simulink model "cursorTask"  (R2012b)
settings: Solver=FixedStepDiscrete  StartTime=0.0  StopTime=10.0  FixedStep=0.001  RelTol=1e-3
undefined symbols (not defined in the file): acquireMethods, autoplayMovementDuration, autoplayReactionTime, autoplayRotationDuration, autoplayRotationStart, centerOffset, clickPercentage, clickRefractoryPeriod, clickTargetColor, clickTargetHoverColor, clickTargs, coherences, contextIDs, contextTime, contextTimeVec, crossSize, cuedText, cuedTextLength, cumulativeDwell, cursorColorClick, cursorColorClosed, cursorColorOpen, cursorColors, cursorDiameter, cursorNeuralColor, cursorNonneuralColor, delayOrder, delayPeriodGainScale, delayTime, discreteOLMode, displayObject, doHeadSpeedFail, drawNumbersOnTargets, dwellRefractoryPeriod, errorAssistAxis, errorAssistR, errorAssistTheta, expRandBinSize, expRandMax, expRandMin, expRandMu, eyeMode, failOnLiftoff, failurePenalty, falseClickFails, fingerPositionTolerance, fixedSeqMode, freePlayMode, gain, gloveBias, gloveLPDenominator, gloveLPNumerator, gloveNonlinearCorrection, gloveXCorrection, gloveYCorrection, gracePeriod, gridEdges, gridSize, gridTilesEachDim, headSpeedCap ... (+134)
(part 2 of 2)

== matlab function cursorTask/cursorTaskSplit ==
  data: xkRaw input double size=[double(xkConstants.NUM_STATE_DIMENSIONS) 1]; xkMod input; behaviorPacket input Bus: behaviorPacketBus size=1; vizData input Bus: peripheralData; clickState input; clickParameters input; taskOutput output Bus: taskOutput; stateParameters input Bus: stateParams size=1; cursorParameters input Bus: taskParamsBus; clock input; xpcTET input; xkModBiasEst input; taskAgnosticXk input; xkAux input
function taskOutput  = cursorTaskCerebus(xkRaw, xkMod, behaviorPacket, vizData, clickState, clickParameters, ...
    stateParameters, cursorParameters, clock, xpcTET, xkModBiasEst, taskAgnosticXk, xkAux)
%#codegen
% This is the state-machine-like implementation of the cursor task. 
% This, depending on paraemters, can do center-out-and-back
%
% October 31 2016: now has two state inputs, xkRaw (which gets fed back to
% the decoder), and xkMod. Generally should look at xkMod for task logic,
% but if the game needs to change a state element which ought to propogate
% into the decoder (for example re-seed the cursor), it should do this to
% both xkRaw and xkMod.

% cursorParameters is actually taskParamsBus, which is set by
% cursotTask_buildWorkspace.m

mouse = behaviorPacket.mouse(1:6);
glove = behaviorPacket.glove(1:5);
robotPosition = behaviorPacket.robotPosition; % 1x3 of x y z % SDS I *think* but need to check that this is the returned position of robot
behaviorRequestClock = behaviorPacket.xpcRequestClock;
peripheralTimestamp = behaviorPacket.peripheralTimestamp(1:16);
%% CONSTANTS
TASK_NAME = 'cursor';
VERSION_ID = single(3.13); % updated to 3.13 with MULTICLICK task -SF
% looking at TASK_DIMS instead of NUM_DIMS to 5D % DIMENSION-DEPENDENT
% NUM_DIMS is dimensionality as the task code was compiled. August 2016 raised this from 2 to 3. Feb 2017 took this to 4
% Actual task can use fewer dimensions, e.g. running 4D with a 5D
% compilation. Look to TASK_DIMS for that. It is defined from locked
% parameters down below
NUM_DIMS = uint8(cursorConstants.NUM_DIMENSIONS); % 
INIT_LENGTH = uint16(100); %ms
% PRE_TRIAL_LENGTH = uint16(20); %ms
SCORE_LENGTH = uint16(4000); %ms
INIT_TIME = uint32(2000);

cursorPosition2 = single( nan(1,NUM_DIMS) ); % Aux cursor and used for RAYS. Can send a second cursor position.
cursorAlpha2 = uint8(100); % used for RAYS, otherwise 100. This is in %.
%% INITIALIZE FILELOGGER DATA
fileLoggerData.data = uint8(zeros(1,1400));
fileLoggerData.dataLen = uint16(0);
fileLoggerData.fileName = uint8(zeros(1,20));
fileLoggerData.send = false;

fileLoggerFormat.format = uint8(zeros(1,1400));
fileLoggerFormat.formatLen = uint16(0);
fileLoggerFormat.fileName = uint8(zeros(1,20));

fileLoggerFormatAndData.format = fileLoggerFormat;
fileLoggerFormatAndData.data = fileLoggerData;
%% INITIALIZE CURSOR TASK OUTPUT - DO NOT REMOVE ANY ASSIGNMENTS, ORDER MATTERS
allowStop = true;
resetHMM = false;

taskOutput.flushFiles = false;
taskOutput.sendFormat = false;
taskOutput.taskDetails = fileLoggerFormat;
taskOutput.discrete = fileLoggerFormatAndData;
taskOutput.continuous = fileLoggerFormatAndData;
taskOutput.screen = fileLoggerFormatAndData;
taskOutput.sound = fileLoggerFormatAndData;
taskOutput.asynch = fileLoggerFormatAndData;
taskOutput.ttl = double(0);
taskOutput.xk = xkRaw;
taskOutput.inputType = cursorParameters.initialInput;
taskOutput.currentTarget = single(zeros([double(xkConstants.NUM_TARGET_DIMENSIONS) 1]));
taskOutput.state = uint16(CursorStates.STATE_INIT);
taskOutput.paused = false;
taskOutput.allowStop = allowStop;
taskOutput.resetHMM = resetHMM;
taskOutput.wiaCode = uint16(1); %garbage
taskOutput.speedCode = uint16(1); %garbage
taskOutput.clickTarget = uint16(DiscreteStates.CLICK_IDLE); 
taskOutput.taskType = uint16(cursorConstants.TASK_CENTER_OUT); %default value -SNF
%% TASK DETAILS PACKET
taskOutput.taskDetails = packFileLoggerTaskDetails(TASK_NAME, VERSION_ID, ...
    'STATE_INIT', uint8(CursorStates.STATE_INIT), ...
    'STATE_PRE_TRIAL', uint8(CursorStates.STATE_PRE_TRIAL),...
    'STATE_NEW_TARGET', uint8(CursorStates.STATE_NEW_TARGET),...
    'STATE_MOVE', uint8(CursorStates.STATE_MOVE),...
    'STATE_ACQUIRE', uint8(CursorStates.STATE_ACQUIRE),...
    'STATE_SUCCESS', uint8(CursorStates.STATE_SUCCESS),...
    'STATE_FAIL', uint8(CursorStates.STATE_FAIL),...
    'STATE_CENTER_TARGET', uint8(CursorStates.STATE_CENTER_TARGET),...
    'STATE_END', uint8(CursorStates.STATE_END),...
    'STATE_RECENTER_DELAY', uint8(CursorStates.STATE_RECENTER_DELAY),...
    'STATE_MOVE_CLICK', uint8(CursorStates.STATE_MOVE_CLICK),...
    'STATE_MOVE_HOVER', uint8(CursorStates.STATE_HOVER),... %SNF: Why in the actual f is this named move_hover and then mapped to just hover??? 
    'STATE_FINGER_MOVED', uint8(CursorStates.STATE_FINGER_MOVED),...
    'CLICK_IDLE', uint8(DiscreteStates.CLICK_IDLE),...
    'CLICK_MAIN', uint8(DiscreteStates.CLICK_MAIN),...
    'TARGET_TYPE_DWELL', uint8(cursorConstants.TARGET_TYPE_DWELL), ...
    'TARGET_TYPE_CLICK', uint8(cursorConstants.TARGET_TYPE_CLICK), ...
    'INPUT_TYPE_MOUSE_ABSOLUTE', uint8(cursorConstants.INPUT_TYPE_MOUSE_ABSOLUTE),...
    'INPUT_TYPE_DECODE_V', uint8(cursorConstants.INPUT_TYPE_DECODE_V),...
    'INPUT_TYPE_AUTO_PLAY', uint8(cursorConstants.INPUT_TYPE_AUTO_PLAY),...
    'CLICK_TYPE_NONE', uint8(clickConstants.CLICK_TYPE_NONE),...
    'CLICK_TYPE_GLOVE', uint8(clickConstants.CLICK_TYPE_GLOVE),...
    'CLICK_TYPE_NEURAL', uint8(clickConstants.CLICK_TYPE_NEURAL),...
    'OUTPUT_TYPE_CURSOR', uint8(cursorConstants.OUTPUT_TYPE_CURSOR),...
    'OUTPUT_TYPE_ROBOT', uint8(cursorConstants.OUTPUT_TYPE_ROBOT)...
);
%% DEFINE PERSISTENTS
persistent state vizPacket;
persistent pauseTriggered;
persistent stateTimer;
persistent holdTimer;
persistent clickTimer; %added SDS Jan 2017, so both click and hold can be used to do this task
persistent cursorColors;
persistent targetRadiusTrans % added SDS Feb 2017, this is the target radius in XYZ
persistent targetRadiusRot % added SDS Feb 2017, this is the target radius in rotation
persistent currentTarget;
persistent nextTarget;
persistent nextClickTarg currentClickTarg; %SNF multiclick
persistent speedCode;
persistent wiaCode;
% below are used for gridlike task, which divides workspace into tiles and
% fails if dwell or click over wrong tile (which makes it a lot like grid
% task. SDS Dec 2016
% D refers to xkConstants.NUM_TARGET_DIMENSIONS, but really not all might
% be used; lockedParams.gridTilesEachDim specifies which dimensions are
% active and how many tiles each dimension is divided into
persistent currentTargetTile; % D x 1 vector of indices into lockedParams.gridEdges. Current active tile I want to go to
persistent nextTargetTile; % D x 1 vector of indices into lockedParams.gridEdges. What the next active target tile will be
persistent currentOccupiedTile; % D x 1 vector of indices specying which tile is currently being occupied.
persistent previousOccupiedTile; % D x 1 vector of indicies specifying which tile was occupied in the previous time step.

persistent currentTargetType nextTargetType;  % dwell or click
persistent trialNum targetOrder cycleNum cycleIndex;
persistent trialDelayLength;

persistent localAcquired localTotal localTotalTime localAcqTime;
persistent localScore totalScore;
persistent acquireTime lastState;

persistent lockedParameters inputType outputType;
persistent stateBeforePreTrial;

persistent lastSoundTime;
persistent lastSoundState;

persistent initialFingerPosition initialCursorPosition previousInput;

persistent totalTaskTime;
persistent lastAcquireSuccess previousTarget;

persistent filteredHeadSpeed;
persistent prevHeadPos;
persistent lastHeadSpeedFail;
%SNF mulitclick: 
persistent prevClickState; 
persistent multiClickColors; 
%% INITIALIZE PERSISTENTS
if(isempty(state))
    state = uint16(CursorStates.STATE_INIT);
    lastState = state;
    currentTarget = single(zeros([double(xkConstants.NUM_TARGET_DIMENSIONS) 1]));
    nextTarget = single(zeros([double(xkConstants.NUM_TARGET_DIMENSIONS) 1]));
    currentTargetTile = uint16(zeros([double(xkConstants.NUM_TARGET_DIMENSIONS) 1])); % SDS Dec 2016
    nextTargetTile = uint16(zeros([double(xkConstants.NUM_TARGET_DIMENSIONS) 1])); % SDS Dec 2016
    currentOccupiedTile = uint16(zeros([double(xkConstants.NUM_TARGET_DIMENSIONS) 1])); % SDS Dec 2016
    previousOccupiedTile = uint16(zeros([double(xkConstants.NUM_TARGET_DIMENSIONS) 1])); % SDS Dec 2016
   
    speedCode = uint16(0); %FRW hacky instructed speed experiment
    wiaCode = uint16(0); %FRW hacky wia experiment
    nextClickTarg = uint16(0);  %SNF for identifying which click target to use
    currentClickTarg = uint16(0);
    
    vizPacket = initVizPacket;
    stateTimer = uint16(0);
    holdTimer = int16(0);
    clickTimer = int16(0); % initialize
    pauseTriggered = true;
    
    cursorColors = double(zeros([3 3])); % there's a second cursor (column 2) allowed; now a third for eye cursor 
    filteredHeadSpeed = single(0);
    prevHeadPos = single(zeros(2,1));

    targetOrder = uint16(ones([1 double(cursorConstants.MAX_TARGETS)]));
    trialNum = uint16(0);
    cycleNum = uint16(0);
    cycleIndex = uint16(1); % 1 so it's a valid idnex even when first used
    trialDelayLength = uint16(0);
    
    localTotal = uint16(0);
    localTotalTime = uint16(0);
    localAcquired = uint16(0);
    localAcqTime = uint16(0);
    localScore = uint16(0);
    totalScore = uint16(0);
    acquireTime = stateTimer;
    currentTargetType = uint16(cursorConstants.TARGET_TYPE_DWELL);
    nextTargetType = uint16(cursorConstants.TARGET_TYPE_DWELL);
	stateBeforePreTrial = uint16(0);
    lastSoundTime = clock;
    lastSoundState = uint8(CursorStates.SOUND_STATE_IDLE);
    
    initialFingerPosition = mouse(1:2);
    initialCursorPosition = single( zeros(NUM_DIMS,1) );
    
    totalTaskTime = uint32(0);
    lastHeadSpeedFail = uint32(0);
    
    lastAcquireSuccess = false;
    previousTarget = currentTarget;
    prevClickState =  uint16(DiscreteStates.CLICK_IDLE); %upon starting, intiialize to not clicking 
        %% buffer all the parameters off the bus
    lockedParameters = cursorParameters;
    targetRadiusTrans = double(lockedParameters.targetDiameter) / 2;
    targetRadiusRot = double(lockedParameters.targetRotDiameter) / 2;
    inputType = lockedParameters.initialInput;
    multiClickColors =  single(lockedParameters.multiclickColors); % single([[255 24 29];[255 0 255]; [140 150 198]; [0 102 255]]); %SNF multiclick- hard coding for now, make this a matrix in task doc
%%
    previousInput = inputType;
end
%% some initialization
if(clock < INIT_TIME)
    pauseTriggered = true;
end
outputType = cursorParameters.outputType; % determines what graphics engine will render this task.
% We usually shouldn't write discrete data
writeDiscreteData = false;
writeContinuousData = true;

if(vizData.receive && (vizData.dataLen > 0 ))
    vizPacket = parseVizPacket(vizData.data);
end

isNeural = (uint16(inputType) == uint16(cursorConstants.INPUT_TYPE_DECODE_V));
%isClicked = (uint16(clickState) == uint16(DiscreteStates.CLICK_MAIN)); %SF: this needs to be more flexible
isClicked = (uint16(clickState) >= uint16(DiscreteStates.CLICK_MAIN)); %SF: this includes multiclick options
isNone = (uint16(inputType) == uint16(cursorConstants.INPUT_TYPE_NONE));
if clickTimer < 0
    clickTimer = clickTimer + 1; %always counts up while negative, thus using up refractory period
end
% clickTimer counts up only in certain states (i.e. only certain states
% allow click accumulation).
if ~isClicked && clickTimer > 0 % doesn't reset to zero when in refractory period.
    clickTimer = int16(0); % resets to be not-clicked
end
%% set the cursor color 
% SNF: add different colors for different clicks in multiclick 
if isClicked
    if uint16(lockedParameters.taskType) == uint16(cursorConstants.TASK_MULTICLICK)
        cursorColors(1:end, 1) = multiClickColors(uint16(clickState-1), 1:end); 
    else
        cursorColors(1:end,1) = lockedParameters.cursorColorClick; %[255; 0; 0;];
    end
elseif isNeural
    cursorColors(1:end,1) = [255; 255; 255;];
elseif isNone
    cursorColors(1:end,1) = [0; 204; 102;];
elseif uint16(inputType) == uint16(cursorConstants.INPUT_TYPE_HEAD_MOUSE)
    cursorColors(1:end,1) = [0; 204; 102;]; %head position is always green
elseif uint16(inputType) == uint16(cursorConstants.INPUT_TYPE_HEAD_CURSORSTILL)
    cursorColors(1:end,1) = [0; 204; 102;]; %primary color represents head position so color it green
else % This is used for autoplay.
    cursorColors(1:end,1) = [255; 255; 255]; % 
%     cursorColors(1:end,1) = [200; 255; 200]; % slightly minty % SDS April 2017: T5 hates minty color, just making it white
end
% these are default colors, individual states can overwrite if they want.
switch lockedParameters.taskType
    case  uint32(cursorConstants.TASK_GRIDLIKE)
        targetColor = 'a'; % in gridlike, target is aqua
    otherwise
        targetColor = 'a'; % in other tasks, target still aqua
end
%% %WIA stuff
if (uint16(lockedParameters.wiaMode) == uint16(cursorConstants.WIA_IMAGINE_ONLY)) || ...
        (uint16(lockedParameters.wiaMode) == uint16(cursorConstants.WIA_IMAGINE_ONLY_NO_HC))
    wiaCode = uint16(2);
elseif uint16(lockedParameters.wiaMode) == uint16(cursorConstants.WIA_WATCH_ONLY)
    wiaCode = uint16(1);
elseif uint16(lockedParameters.wiaMode) == uint16(cursorConstants.WIA_DO_ONLY)
    wiaCode = uint16(3);
end
%% which state elements do I look to for the cursor's position? SDS July 2016
xk2HorizontalPos = uint8( lockedParameters.xk2HorizontalPos );
xk2VerticalPos = uint8( lockedParameters.xk2VerticalPos );
xk2HorizontalVel = uint8( lockedParameters.xk2HorizontalVel );
xk2VerticalVel = uint8( lockedParameters.xk2VerticalVel );
xk2DepthPos = uint8( lockedParameters.xk2DepthPos );
xk2DepthVel = uint8( lockedParameters.xk2DepthVel );
xk2RotatePos = uint8( lockedParameters.xk2RotatePos );
xk2RotateVel = uint8( lockedParameters.xk2RotateVel );
xk2Rotate2Pos = uint8( lockedParameters.xk2Rotate2Pos );
xk2Rotate2Vel = uint8( lockedParameters.xk2Rotate2Vel );
% DIMENSION-DEPENDENT
TASK_DIMS = lockedParameters.numDisplayDims; % only used for determining what kind of
% checking to use. We still need to have everything be NUM_DIMS long or
% things won't compile.
canBePosInds = [xk2HorizontalPos,xk2VerticalPos,xk2DepthPos,xk2RotatePos,xk2Rotate2Pos];
canBeVelInds = [xk2HorizontalVel,xk2VerticalVel,xk2DepthVel,xk2RotateVel,xk2Rotate2Vel];
effectorPosInds = canBePosInds(1:NUM_DIMS);
effectorVelInds = canBeVelInds(1:NUM_DIMS);

if uint16(inputType) == uint16(cursorConstants.INPUT_TYPE_HEAD_CURSORSTILL)
    effectorPos = xkAux(effectorPosInds);
    effectorVel = xkAux(effectorVelInds);
    auxEffectorPos = xkMod(effectorPosInds);
    displayAuxCursor = true;
    cursorColors(1:end,2) = [255; 255; 255];
elseif uint16(inputType) == uint16(cursorConstants.INPUT_TYPE_CURSOR_HEADSTILL) || ...
        uint16(inputType) == uint16(cursorConstants.INPUT_TYPE_AUTO_ACQUIRE_HS)
    effectorPos = xkMod(effectorPosInds);
    effectorVel = xkMod(effectorVelInds);
    auxEffectorPos = xkAux(effectorPosInds);
    displayAuxCursor = true;
    cursorColors(1:end,2) = [0; 204; 102;];
elseif uint16(inputType) == uint16(cursorConstants.INPUT_TYPE_CURSOR_AND_HEAD)
    effectorPos = xkMod(effectorPosInds);
    effectorVel = xkMod(effectorVelInds);
    %for target acquisiotn logic, the 3rd and 4th dimensions of the cursor
    %will be equal to auxiliary cursor X and Y and the task will be 4-dimensional
    effectorPos(3:4) = xkAux(effectorPosInds(1:2));
    effectorVel(3:4) = xkAux(effectorVelInds(1:2));
    auxEffectorPos = xkAux(effectorPosInds);
    displayAuxCursor = true;
    cursorColors(1:end,2) = [0; 204; 102;];
elseif uint16(inputType) == uint16(cursorConstants.INPUT_TYPE_WIA_HEAD)
    if wiaCode==uint16(1) || wiaCode==uint16(2) %watch, imagine
        effectorPos = xkMod(effectorPosInds);
        effectorVel = xkMod(effectorVelInds);
        auxEffectorPos = xkAux(effectorPosInds);
        if (uint16(lockedParameters.wiaMode) == uint16(cursorConstants.WIA_IMAGINE_ONLY_NO_HC))
            displayAuxCursor = false;
        else
            displayAuxCursor = true;
        end
        cursorColors(1:end,2) = [0; 204; 102;];
    else %attempt
        effectorPos = xkAux(effectorPosInds);
        effectorVel = xkAux(effectorVelInds);
        auxEffectorPos = xkMod(effectorPosInds);
        displayAuxCursor = false;
        cursorColors(1:end,1) = [0; 204; 102;];
    end
else
    effectorPos = xkMod(effectorPosInds);
    effectorVel = xkMod(effectorVelInds);
    auxEffectorPos = zeros(NUM_DIMS,1);
    displayAuxCursor = false;
end
%% %head speed check; we low pass filter the 1ms head speed and can fail the trial if it is too high
headSpeedAlpha = single(0.96);
headSpeed = 1000*sqrt(sum((behaviorPacket.windowsMousePosition - prevHeadPos).^2));
filteredHeadSpeed = headSpeedAlpha*filteredHeadSpeed + (1-headSpeedAlpha)*headSpeed;
prevHeadPos = behaviorPacket.windowsMousePosition;
%fail if moving the head when he shouldn't be
if (lockedParameters.doHeadSpeedFail || wiaCode==uint16(1) || wiaCode==uint16(2)) && (filteredHeadSpeed > lockedParameters.headSpeedCap) ...
    &&((clock - lastHeadSpeedFail)>2000)
    %stateTimer = uint16(0);
    %state = uint16(CursorStates.STATE_FAIL);
    lastHeadSpeedFail = clock;
    lastSoundTime = clock;
    lastSoundState = uint8(CursorStates.SOUND_STATE_FAIL);
end
%% %really hacky eye mode
eyePos = behaviorPacket.windowsPC1GazePoint;
eyePos(1) = (eyePos(1)-0.5)*1680;
eyePos(2) = (eyePos(2)-0.5)*1050;
cursorPosition3 = single(nan(NUM_DIMS,1));
if lockedParameters.eyeMode==1
    effectorPos(1:2) = eyePos;
    cursorColors(1:end,1) = [255; 133; 0;];
elseif lockedParameters.eyeMode==2
    auxEffectorPos(1:2) = eyePos;
elseif lockedParameters.eyeMode==3
    cursorColors(1:end,3) = [255; 133; 0;];
    cursorPosition3(1:NUM_DIMS) = 0;
    cursorPosition3(1:2) = eyePos;
end
%% free play mode
if cursorParameters.freePlayMode==uint16(1)
    state = uint16(CursorStates.STATE_INIT);
    stateTimer = uint16(0);
end
%% holding-still checks: 
%--the auxiliary cursor must be in the center to acquire a target with the actual cursor
%--in modes where the aux. cursor is not used, its position is zero, placing
%  it in the center so it will pass all auxInCenter checks
auxInCenter = sqrt(sum(auxEffectorPos.^2))<80;
if (uint16(inputType) == uint16(cursorConstants.INPUT_TYPE_CURSOR_AND_HEAD)) || ...
        lockedParameters.speedTaskMode==1 || wiaCode==uint16(3) || ...
        (uint16(lockedParameters.wiaMode) == uint16(cursorConstants.WIA_IMAGINE_ONLY_NO_HC))
    auxInCenter = true; %don't check for aux cursor in center for dual effector mode
end
%display auxiliary cursor
if displayAuxCursor
    cursorPosition2 = single(auxEffectorPos);
end
%% fingerlifted is set when finger comes off the touchpad - UNUSED SNF
fingerLifted = (mouse(3)==0);
fingerOffTarget = sqrt(sum((double(initialFingerPosition)-double(mouse(1:2))).^2)) > double(lockedParameters.fingerPositionTolerance) || mouse(3) ==0;
if ~pauseTriggered
    totalTaskTime = totalTaskTime+1;
end
%% generally, allow cursor to stop off target. check options
allowStop = lockedParameters.stopOffTarget;

if clock> INIT_TIME && state~= uint16(CursorStates.STATE_INIT) && state ~= uint16(CursorStates.STATE_CENTER_TARGET) ...
        && state ~= uint16(CursorStates.STATE_FINGER_MOVED) ...
        && lockedParameters.lockFingerPosition && fingerOffTarget
    % Game is locked awaiting finger liftoff. Old stuff that Chethan/Paul
    % wrote, I don't know what it really does or why. -Sergey
    previousInput = inputType;
    inputType = uint16(cursorConstants.INPUT_TYPE_MOUSE_ABSOLUTE);
    state = uint16(CursorStates.STATE_FINGER_MOVED);
    cursorColors(1:end,1) = [255;133;0];
    stateTimer = uint16(0);
    currentTarget(1:NUM_DIMS,:) = single(initialCursorPosition); 
else
%% %%%%%%%%%%%%%%%%%%%%%%%%%%%%%%%%%%%%%%%%%%%%%%%%%%%%%%%%%%%%%%%%%%%% 
%%%   STATE MACHINE IMPLEMENTATION
%%%%%%%%%%%%%%%%%%%%%%%%%%%%%%%%%%%%%%%%%%%%%%%%%%%%%%%%%%%%%%%%%%%%%%%%
    switch state
%% STATE_INIT
        case {CursorStates.STATE_INIT}
            % set all the persistents that may have been changed by user input
            pauseTriggered = stateParameters.pause;
            lockedParameters = cursorParameters;
            writeContinuousData = false;
            inputType = lockedParameters.initialInput;
            % generate some entropy
            jnk = rand(1,1);
            initialFingerPosition = mouse(1:2);
%             initialCursorPosition = xkMod(canBePosInds(1:NUM_DIMS)); % handhold the compiler so it knows its fixed dim.
            initialCursorPosition = single( zeros(NUM_DIMS,1) );
            if ~pauseTriggered
                stateTimer = stateTimer + 1;
            end
            if stateTimer >= INIT_LENGTH
                stateTimer = uint16(0);
                trialNum = uint16(0);
                currentTarget(:) = single(zeros(double(xkConstants.NUM_TARGET_DIMENSIONS),1)); 
                cycleNum = uint16(0);
                % Different first state (after INIT) depending on the task. SDS Dec 2016
                switch lockedParameters.taskType
                    case  uint32(cursorConstants.TASK_GRIDLIKE)
                        % For gridlike task, go straight to generating a new target.
                       % state = uint16(CursorStates.STATE_PRE_TRIAL);
                    case uint32(cursorConstants.TASK_RANDOM)
                        % same for Random task.
                       % state = uint16(CursorStates.STATE_PRE_TRIAL);
                    case {uint32(cursorConstants.TASK_RAYS), ...
                            uint32(cursorConstants.TASK_CENTER_OUT_NO_BACK), ...
                            uint32(cursorConstants.TASK_FCC)}
                        % need to have some initial target order since we
                        % don't start with 0 being active target which is
                        % easy to acquire to start the chain
                        currentTarget(1:end) = 9999; % start with target off-screen
                       % state = uint16(CursorStates.STATE_PRE_TRIAL);%                        
                    otherwise
%                         state = uint16(CursorStates.STATE_CENTER_TARGET);
                       % state = uint16(CursorStates.STATE_PRE_TRIAL); % SDS Mar 27 2017, why not start here?
                        % give an initial targetOrder (for variants like
                        % TASK_CENTER_OUT) so that even if first trial is a
                        % failure. there's a target order to give it after
                        % next center success
                        targetOrder(1:lockedParameters.numTargets) = randperm(lockedParameters.numTargets);
                end
                % all of these go to PRE_TRIAL, as they should. Moved out here:
                state = uint16(CursorStates.STATE_PRE_TRIAL); % SNF: all tasks go INIT-> PRE_TRIAL. 
            end
%% STATE_PRE_TRIAL            
        case {CursorStates.STATE_PRE_TRIAL}
            %% capture pauses
            if stateTimer == 0
                pauseTriggered = stateParameters.pause;
                stateBeforePreTrial = lastState;
            end
            if ~pauseTriggered
                stateTimer = stateTimer + 1;
            end
            % don't do this on 0, because if we're paused, 0 will occur many many times
            if stateTimer == 1
                %% choose the next target. Here's where it comes in from task parameters bus
                lockedParameters = cursorParameters;
                % This is the unintuitive place where click is actually set
                % as the nextTargetType, which is then propogated to
                % currentTargetType. I guess at some point they could
                % randomize click or hold trials?
                clickRand = rand(1,1);
                if clickRand < lockedParameters.clickPercentage && stateBeforePreTrial ~= uint16(CursorStates.STATE_SCORE_TARGET)
                    nextTargetType = uint16(cursorConstants.TARGET_TYPE_CLICK);
                else
                    nextTargetType = uint16(cursorConstants.TARGET_TYPE_DWELL);
                end %SNF moved this up here so it can be overwritten by MULTITASK. 
                
                targetRadiusTrans = double(lockedParameters.targetDiameter) / 2; %this is the same everywhere except random. SNF moved it.
                targetRadiusRot = double(lockedParameters.targetRotDiameter) / 2; %this is the same everywhere except random. SNF moved it.
                %SNF: add this so this field is always populated: 
                nextClickTarg = uint16(DiscreteStates.CLICK_IDLE);%SNF for backwards compatibility
                switch lockedParameters.taskType % DIFFERENT TARGET CHOOSING RULES DEPENDING ON THE TASK TYPE.
                    case uint32(cursorConstants.TASK_CENTER_OUT)
                       if mod(trialNum, 2) == 0 
                            % CENTER TARGET - the center target is "special" and is set here.
                            nextTarget = single(zeros( double( xkConstants.NUM_TARGET_DIMENSIONS ), 1) );
                            %nextClickTarg = uint16(DiscreteStates.CLICK_IDLE);%SNF for backwards compatibility
                        else
                            % OTHER TARGETS - The other targets come from lockedParameters.targetInds.                               
                            nextTarget = lockedParameters.targetInds(:,targetOrder(cycleIndex));
                            nextClickTarg = uint16(DiscreteStates.CLICK_MAIN); %SNF: for backwards compatibility 
                        end
%                         targetRadiusTrans = double(lockedParameters.targetDiameter) / 2;
%                         targetRadiusRot = double(lockedParameters.targetRotDiameter) / 2;               
                    case uint32(cursorConstants.TASK_MULTICLICK)
                        if mod(trialNum, 2) == 0 % CENTER TARGET is "special" and is set here.
                            nextTarget = single(zeros( double( xkConstants.NUM_TARGET_DIMENSIONS ), 1) );
                            nextTargetType = uint16(cursorConstants.TARGET_TYPE_DWELL);
                            nextClickTarg = uint16(0); %indicates no background image 
                        else % OTHER TARGETS come from lockedParameters.targetInds.                              
                            nextTarget = lockedParameters.targetInds(:,targetOrder(cycleIndex));
                            nextTargetType = uint16(cursorConstants.TARGET_TYPE_CLICK); %SNF multiclick, distinguishes from dwell 
                            nextClickTarg = lockedParameters.clickTargs(targetOrder(cycleIndex)); 
                        end
                      %  targetRadiusTrans = double(lockedParameters.targetDiameter) / 2;
                      %  targetRadiusRot = double(lockedParameters.targetRotDiameter) / 2;
                    case uint32( cursorConstants.TASK_CENTER_OUT_NO_BACK )
                        nextTarget = lockedParameters.targetInds(:,targetOrder(cycleIndex));
                        %% reset cursor to center
                        xkMod([effectorPosInds,effectorVelInds],1) = 0;
                        % also do this to xkRaw
                        xkRaw([effectorPosInds,effectorVelInds],1) = 0;
                        %These tasks don't alternate like center out and back- 
                        %if they dwell, they won't go to HOVER and this won't matter in getClickState 
                        nextClickTarg = uint16(DiscreteStates.CLICK_MAIN); %SNF: for backwards compatibility 
%                         targetRadiusTrans = double(lockedParameters.targetDiameter) / 2;
%                         targetRadiusRot = double(lockedParameters.targetRotDiameter) / 2;
                    case { uint32( cursorConstants.TASK_RAYS ), ...
                            uint32( cursorConstants.TASK_FCC ) }
                        % Fully random selection of next target
                        cycleIndex = uint16( randperm(lockedParameters.numTargets,1) );
                        nextTarget = lockedParameters.targetInds(:,cycleIndex);
                        %These tasks don't alternate like center out and back- 
                        %if they dwell, they won't go to HOVER and this won't matter in getClickState 
                        nextClickTarg = uint16(DiscreteStates.CLICK_MAIN); %SNF: for backwards compatibility 
%                         targetRadiusTrans = double(lockedParameters.targetDiameter) / 2;
%                         targetRadiusRot = double(lockedParameters.targetRotDiameter) / 2;
                    case uint32( cursorConstants.TASK_PINBALL )                   
                        nextTarget = lockedParameters.targetInds(:,targetOrder(cycleIndex));
%                         targetRadiusTrans = double(lockedParameters.targetDiameter) / 2;
%                         targetRadiusRot = double(lockedParameters.targetRotDiameter) / 2;
                        %These tasks don't alternate like center out and back- 
                        %if they dwell, they won't go to HOVER and this won't matter in getClickState 
                        nextClickTarg = uint16(DiscreteStates.CLICK_MAIN); %SNF: for backwards compatibility 
                    case uint32( cursorConstants.TASK_RANDOM )
                        % SDS Mar 2017. Randomly choose a target location
                        % from within the workspace boundaries and a target
                        % size as a multiple of randomTaskSizeMultipliers.
                        % If the workspace of a dimension is zero, it'll
                        % set that target coordinate to zero as well.
                        randRolls = rand(TASK_DIMS,1); % uniform 0 to 1 
                        for iDim = 1 : TASK_DIMS
                            myRange = lockedParameters.randomTaskBoundaries(iDim,1:2);
                            nextTarget(iDim) = myRange(1) + randRolls(iDim)*(myRange(2)-myRange(1));
                        end
                        %These tasks don't alternate like center out and back- 
                        %if they dwell, they won't go to HOVER and this won't matter in getClickState 
                        nextClickTarg = uint16(DiscreteStates.CLICK_MAIN); %SNF: for backwards compatibility 
                        % determine the target diameter. Note it uses same
                        % index for randomTaskTargetDiameters and randomTaskTargetRotDiameters
                        % under the assumption that even if these aren't
                        % identical (they nromally will be identical),
                        % they're at least matched and in the same order.
                        % This gives us the capability fo amking rotation
                        % across-the-board easier by e.g. having ti always
                        % be slightly alrger that xyz diameters
                        chooseSize = randperm(  min(nnz(lockedParameters.randomTaskTargetDiameters), double(cursorConstants.MAX_DIAMETERS) ) ); % min is to bound memory size to handhold compiler
                        chooseSize = chooseSize(1);
                        targetRadiusTrans =  double( lockedParameters.randomTaskTargetDiameters(chooseSize) )/2;
                        targetRadiusRot = double( lockedParameters.randomTaskTargetRotDiameters(chooseSize) )/2;
                    case  uint32(cursorConstants.TASK_GRIDLIKE)
                        % SDS Dec 2016 TODO: Set the translational radius based on spacing of tiles.
%                         targetRadiusTrans = double(lockedParameters.targetDiameter) / 2;
%                         targetRadiusRot = double(lockedParameters.targetRotDiameter) / 2;
                        % randomly choose a tile                                                
                        for iDim = 1 : numel( lockedParameters.gridTilesEachDim )
                           if lockedParameters.gridTilesEachDim(iDim) > 0 
                              %this is an active dimension 
                              randOrder = randperm(lockedParameters.gridTilesEachDim(iDim) );
                              myTile = randOrder(1);
                              nextTargetTile(iDim) = myTile; % take the first one (randomize)
                              % now that we have the targetTile, I can look  at gridEdges to get center of this tile in this dimension
                              nextTarget(iDim) = 0.5*( lockedParameters.gridEdges(myTile,iDim) + lockedParameters.gridEdges(myTile+1,iDim) );
                           %else
                               % do nothing, nextTarget(iDim) stays how it was initialized, presumably 0
                           end
                        end
                        %These tasks don't alternate like center out and back- 
                        %if they dwell, they won't go to HOVER and this won't matter in getClickState 
                        nextClickTarg = uint16(DiscreteStates.CLICK_MAIN); %SNF: for backwards compatibility 
                end                
                %hacky instructed speed experiment FRW
                if (lockedParameters.speedTaskMode==2)
                    %only change code on an outer target
                    if ~all(nextTarget==0)
                        speedCode = uint16(randi(3));
                    end
                end
                
                % hacky WIA experiment FRW
                if uint16(lockedParameters.wiaMode)==uint16(cursorConstants.WIA_WATCH_IMAGINE_ATTEMPT)
                    if ~all(nextTarget==0)
                        wiaCode = uint16(randi(3));
                    end
                end
% write the discrete data once per trial with all these values we just set
                writeDiscreteData = true;                
            end
            
            if lockedParameters.taskType == uint32( cursorConstants.TASK_RAYS )
                % color target to show if preceding trial was success or
                % failure                
                if lastAcquireSuccess
                    targetColor = 'g';
                else
                    targetColor = 'r';
                end
                % lock cursor at zero during this.
                % reset cursor to center
                xkMod([effectorPosInds,effectorVelInds],1) = 0;
                % also do this to xkRaw
                xkRaw([effectorPosInds,effectorVelInds],1) = 0;
            end
            
            if stateTimer >= lockedParameters.preTrialLength;
                stateTimer = uint16(0);
                if trialNum > lockedParameters.numTrials
                    %% are we done?
                    state = uint16(CursorStates.STATE_END);
                else
                    state = uint16(CursorStates.STATE_NEW_TARGET);
                end               
                trialDelayLength = uint16(0);                
            end     
%% STATE_NEW_TARGET
        case {CursorStates.STATE_NEW_TARGET}
            % for both timers, don't reset to 0 if they're negative (don't
            % automatically burn up the refractory period).
            clickTimer = int16(0); % no accumulating click during thhis state, and its reset to 0
            if ~trialDelayLength && ~all(nextTarget==0)
                if lockedParameters.useRandomDelay
                    % pick a new random delay
                    while double(trialDelayLength) < lockedParameters.expRandMin || double(trialDelayLength) > lockedParameters.expRandMax
                        trialDelayLength = uint16(lockedParameters.expRandMu * -log(rand([1 1])));
                    end
                    trialDelayLength = uint16(round(double(trialDelayLength) / double(lockedParameters.expRandBinSize))*lockedParameters.expRandBinSize);
                else
                    trialDelayLength = uint16(lockedParameters.expRandMu);
                end
            end
            % Check whether cursor is in target differs for Gridlike task.
             %SNF : THIS SHOULD BE AN IF STATEMENT, YA HEATHENS
            switch lockedParameters.taskType
                case uint32( cursorConstants.TASK_GRIDLIKE )
                    myTile = whichGridlikeTile( effectorPos, lockedParameters.gridEdges, lockedParameters.gridTilesEachDim );
                    cursorOnTarget = ~any( myTile ~= currentTargetTile ); % SDS Dec 2016          
                    % refractory period  happens here. Effectively, you get this much extra time after
                    holdTimer = -int16( lockedParameters.selectionRefractoryMS );  
                otherwise
                    cursorOnTarget =  isCursorOnTarget(effectorPos, double(lockedParameters.cursorDiameter)/2, currentTarget, targetRadiusTrans, double( targetRadiusRot ), TASK_DIMS);
            end
            
            stateTimer = stateTimer + 1;
            if stateTimer >= trialDelayLength
                % great, present the new target now
                stateTimer = uint16(0);
                previousTarget = currentTarget;
                currentTarget = nextTarget;
                currentTargetType = nextTargetType;                
                currentClickTarg = nextClickTarg; % SNF this happens *AFTER* writing discrete data
                
                if holdTimer < 0
                    holdTimer = int16(0); % reset hold timer. Needed now for Gridlike task logic SDS 15 Dec 2016
                end
                % click refractory period applied  here.
                clickTimer = -int16( lockedParameters.selectionRefractoryMS );
                % If this is gridlike task, also update the currentTargetTile
                if lockedParameters.taskType == uint32(cursorConstants.TASK_GRIDLIKE)
                    currentTargetTile = nextTargetTile;
                    % should I also change current and prevous
                    % OccupiedTile? I think probably not..
                end
                % is recentering turned on, and does that apply here?
                if (lockedParameters.recenterOnSuccess  && lastAcquireSuccess == true ) || ...
                   (lockedParameters.recenterOnFail     && lastAcquireSuccess == false)
                    recenterThisTrial = true;
                else
                    recenterThisTrial = false;
                end             
                
                if recenterThisTrial
                    stateTimer = uint16(0);
                    state = uint16(CursorStates.STATE_RECENTER_DELAY);
                else
                    if lockedParameters.soundOnGo
                        lastSoundTime = clock;
                        lastSoundState = uint8(CursorStates.SOUND_STATE_GO);
                    end
                    % Key logic for whether to go into STATE_MOVE or
                    % STATE_MOVE_CLICK, based on what mode is selected,
                    if currentTargetType == cursorConstants.TARGET_TYPE_CLICK;
                        state = uint16(CursorStates.STATE_MOVE_CLICK);
                    elseif currentTargetType == cursorConstants.TARGET_TYPE_DWELL;
                        state = uint16(CursorStates.STATE_MOVE);
                    end
                end
            elseif ~cursorOnTarget && lockedParameters.taskType ~= uint32(cursorConstants.TASK_GRIDLIKE) && ...
                    uint16(lockedParameters.wiaMode)~=uint16(cursorConstants.WIA_IMAGINE_ONLY_NO_HC)
                %fail if cursor moves outside target region during delay
                %period (except during WIA imagine mode, where the autoplay
                %cursor is invisible and is just used to make the task
                %proceed with a certain cadence)
                stateTimer = uint16(0);
                state = uint16(CursorStates.STATE_FAIL);
                %lastSoundTime = clock;
                %lastSoundState = uint8(CursorStates.SOUND_STATE_FAIL);
            end            
%% STATE_RECENTER_DELAY
        case {CursorStates.STATE_RECENTER_DELAY}
            % (Gridlike and Random task variants never enters this state)
            stateTimer = stateTimer + 1;
            if stateTimer <= lockedParameters.recenterDelay
                switch lockedParameters.taskType
                    case {uint32( cursorConstants.TASK_PINBALL ), ...
                            uint32(cursorConstants.TASK_CENTER_OUT), ...
                            uint32(cursorConstants.TASK_GRIDLIKE),...
                            uint32(cursorConstants.TASK_RANDOM)}
                        xkMod(effectorPosInds,1) = previousTarget(1:NUM_DIMS);
                        xkRaw(effectorPosInds,1) = previousTarget(1:NUM_DIMS);
                        xkMod(effectorVelInds,1) = 0;
                        xkRaw(effectorVelInds,1) = 0;
                    case  uint32(cursorConstants.TASK_MULTICLICK) %SNF multiclick task
                        xkMod(effectorPosInds,1) = 0;
                        xkRaw(effectorPosInds,1) = 0;
                        xkMod(effectorVelInds,1) = 0;
                        xkRaw(effectorVelInds,1) = 0;     
                    case uint32( cursorConstants.TASK_CENTER_OUT_NO_BACK )
                        xkMod([effectorPosInds, effectorVelInds],1) = 0;
                        xkRaw([effectorPosInds, effectorVelInds],1) = 0;
                    case uint32( cursorConstants.TASK_RAYS )
                        xkMod([effectorPosInds, effectorVelInds],1) = 0;
                        xkRaw([effectorPosInds, effectorVelInds],1) = 0;
                end
            else %if the recenter delay has elapsed 
                if lockedParameters.soundOnGo
                    lastSoundTime = clock;
                    lastSoundState = uint8(CursorStates.SOUND_STATE_GO);
                end
                stateTimer = uint16(0);
%                 if lockedParameters.taskType == uint32(cursorConstants.TASK_MULTICLICK) %SNF multiclick task
%                     % this state is only entered into if the peripheral
%                     % target failed, so basically skip the center target
% %                     if currentTargetType == cursorConstants.TARGET_TYPE_CLICK;
% %                         state = uint16(CursorStates.STATE_MOVE_CLICK);
% %                     else %only recenter if the next target is the center
%                         state = uint16(CursorStates.STATE_SUCCESS);
%                    % end
                %elseif currentTargetType == cursorConstants.TARGET_TYPE_CLICK;
                if currentTargetType == cursorConstants.TARGET_TYPE_CLICK
                    state = uint16(CursorStates.STATE_MOVE_CLICK);
                elseif currentTargetType == cursorConstants.TARGET_TYPE_DWELL
                    if lockedParameters.taskType == uint32(cursorConstants.TASK_MULTICLICK)
                        state = uint16(CursorStates.STATE_SUCCESS);
                    else
                        state = uint16(CursorStates.STATE_MOVE);
                    end
                end                
                % reset click timer after leaving this state as well, but
                % don't zero the refractory period if it's still negative.
                % Note that beign in this state does use up refractory click period.
                if clickTimer > 0
                    clickTimer = int16(0);
                end
            end            
%% STATE_MOVE            
        case {CursorStates.STATE_MOVE}
            stateTimer = stateTimer + 1;
            inputType = lockedParameters.inputType; % needed to unlock cursor if not coming from success state
            % Check whether cursor is in target differs for Gridlike task.
            switch lockedParameters.taskType
                case uint32( cursorConstants.TASK_GRIDLIKE )
                    currentOccupiedTile = whichGridlikeTile( effectorPos, lockedParameters.gridEdges, lockedParameters.gridTilesEachDim );
                    cursorOnTarget = ~any( currentOccupiedTile ~= currentTargetTile ); % SDS Dec 2016
                    translateOnTarget = false; % just so it is defined.
                case uint32( cursorConstants.TASK_RAYS )
                    % SPECIAL RAYS LOGIC                
                    translateOnTarget = false; % not used
                    cursorOnTarget = false;% avoids the usual logic below.
                    % uses function defined at bottom.
                    currentTargetInd = cycleIndex; % using cycleIndex for this,
                    % but note targets are random and therefore it's not
                    % really a cycle.
                    [selectionHappens, cursorOnCorrectTarget, closestTargetInd] = RAYSselection(effectorPos, double(lockedParameters.targetRotDiameter)/2, currentTargetInd, ...
                        lockedParameters.targetInds, lockedParameters.numTargets, TASK_DIMS);
                    % send coordinates of currently selected target over to
                    % viz computer.
                    if ~cursorOnCorrectTarget
                        % uncomment below to show closest target
%                         cursorPosition2(1:end) = single( lockedParameters.targetInds(:,closestTargetInd) );
                        % cursor2 alpha depends on how close cursor is to
                        % decision boundary.   
                        top = norm(effectorPos);
                        bottom = norm(double(lockedParameters.targetRotDiameter)/2);
                        cursorAlpha2 = uint8(100*top/bottom );
                        % Cursor2 shows projection of cursor position onto
                        % the target shell.
                        distToShell = norm( lockedParameters.targetInds(:,1) );
                        cursorPosition2(1:end) = single( distToShell.*effectorPos./norm(effectorPos) );
                    else
                       % color the target orange
                       targetColor = 'o';
                    end
                    
                    if selectionHappens
                        % OK, trial ends one way or the other
                        if cursorOnCorrectTarget
                            % Success
                            acquireTime = stateTimer;
                            stateTimer = uint16(0);
                            state = uint16(CursorStates.STATE_SUCCESS);
                            targetColor = 'g';
                        else
                            %failure
                            stateTimer = uint16(0);
                            state = uint16(CursorStates.STATE_FAIL);   
                            % move the target to what was erroneously
                            % selected.
                            currentTarget = lockedParameters.targetInds(:,closestTargetInd);
                            targetColor = 'r';
                        end
                    end
                    
                % If we want a dwell TASK_FCC, need to implement target-specific counteing here like what is done for GRIDLIKE
                otherwise
                    [cursorOnTarget, translateOnTarget] = isCursorOnTarget(effectorPos, double(lockedParameters.cursorDiameter)/2, currentTarget, targetRadiusTrans, targetRadiusRot, TASK_DIMS);
            end
            
            if translateOnTarget && lockedParameters.numDisplayDims > 3
                targetColor = 'n'; % special, tells the graphics to show that cursor is
                % translated currectly but not yet rotated correctly;
                % doesn't happen in RAYS regardless.
            end            
            
            if cursorOnTarget && auxInCenter
                state = uint16(CursorStates.STATE_ACQUIRE);
                if holdTimer >= 0
                    holdTimer = int16(0); % reset hold timer -- it could have been nonzero from either previous
                    % target hold or time spent in any tile in Gridlike mode.
                else
                    holdTimer = holdTimer; % allows negative to carry over for selectionRefractoryMS
                end
                
                if lockedParameters.soundOnOverTarget
                    % if we're on autoplay, make a tapping noise
                    lastSoundTime = clock;
                    lastSoundState = uint8(CursorStates.SOUND_STATE_OVER_TARGET);
                end
                
            elseif stateTimer >= lockedParameters.trialTimeout
                stateTimer = uint16(0);
                state = uint16(CursorStates.STATE_FAIL);
           
            elseif lockedParameters.failOnLiftoff && fingerLifted
                stateTimer = uint16(0);
                state = uint16(CursorStates.STATE_FINGER_LIFTED);
          
            elseif lockedParameters.taskType ==  uint32(cursorConstants.TASK_GRIDLIKE)
                % GRIDLIKE TASK COUNTING OF TIME SPENT IN WRONG TILE
                % SDS Dec 2016                
                if any( currentOccupiedTile)  % to rule out being in no tile
                    if any( currentOccupiedTile ~= previousOccupiedTile )
                        % Entered a new tile - reset timer
                        if holdTimer >= 0
                            holdTimer = int16(0);
                        else
                            holdTimer = holdTimer;
                           % allows negative holdTimer to carry over for selectionRefractoryMS 
                        end
                    else
                        holdTimer = holdTimer + 1;
                        % still in the same tile as before, so count count up hold timer
                        if holdTimer > lockedParameters.holdTime
                            % dwelled too long in wrong tile; FAIL!
                            stateTimer = uint16(0);
                            state = uint16(CursorStates.STATE_FAIL);
                        end
                    end
                else
                   % can count up from negative to 0 (being outside of bounday still counts towards grace period.
                   if holdTimer < 0
                       holdTimer = holdTimer + 1;
                   end
                end
            end
            % for Gridlike task (Irrelevant otherwiseen). End of state,
            % previous tile is set to current tile. SDS Dec 2016
            previousOccupiedTile = currentOccupiedTile; 
%% STATE_FINGER_LIFTED
        % Not currently used - SDS Dec 2016
        case {CursorStates.STATE_FINGER_LIFTED}
            stateTimer = stateTimer + 1;
            if ~fingerLifted
                stateTimer = uint16(0);
                state = uint16(CursorStates.STATE_FAIL);
            end
%% STATE_MOVE_CLICK
        case {CursorStates.STATE_MOVE_CLICK}           
            stateTimer = stateTimer + 1;
            inputType = lockedParameters.inputType; % needed to unlock if not coming from success
            % Click accumulation happens here.
           % if clickState == uint16(DiscreteStates.CLICK_MAIN)
            if clickState >= uint16(DiscreteStates.CLICK_MAIN) %SNF to include multiclick states... this might mess with idle
            %SNF: this needs to include logic for if the previous click is
            %the same as the current click, logic which totally should be
            %handled by discreteDecode/HMMStateDecoder but putting a
            %comment paragraph here just in case. lol @ readability of code
            % SNF: if you're coming from the idle state *or* the same click, increment the clickTimer
                if (prevClickState ==  uint16(DiscreteStates.CLICK_IDLE)) || (uint16(clickState) == prevClickState)
                    clickTimer = clickTimer + 1; 
                else %otherwise, reset. 
                    clickTimer = int16(0); 
                end
            end
            % Recall that resetting of this timer happens
            % if not clicking happens at top of this function call, i.e. regardless of state            
            networkOutput.discrete.send = false; % SDS: not really sure why this is set here but not in e.g. STATE_MOVE
            % Check whether cursor is in target differs for Gridlike task.
            switch lockedParameters.taskType
                case  uint32(cursorConstants.TASK_GRIDLIKE)
                    currentOccupiedTile = whichGridlikeTile( effectorPos, lockedParameters.gridEdges, lockedParameters.gridTilesEachDim );
                    cursorOnTarget = ~any( currentOccupiedTile ~= currentTargetTile ); % SDS Dec 2016
                    targetColor = 'a'; % in gridlike task, color is aqua (but if we're over target, it'll change)
                    translateOnTarget = false; % just so it is defined. TODO: make so it is useful 
              
                case uint32( cursorConstants.TASK_FCC )
                    [cursorOnTarget, closestTargetInd] = FCCisCursorOntarget(effectorPos, cycleIndex, ...
                        lockedParameters.targetInds, lockedParameters.numTargets, TASK_DIMS );
                    % closestTargetInd not yet used but could be for
                    % selecting specific letters.
                    translateOnTarget = false; % must be defined, but not used
                otherwise
                    [cursorOnTarget, translateOnTarget] = isCursorOnTarget(effectorPos, double(lockedParameters.cursorDiameter)/2, currentTarget, targetRadiusTrans, targetRadiusRot, TASK_DIMS);
                    targetColor = 'a';
            end
            
            if translateOnTarget && lockedParameters.numDisplayDims > 3
                targetColor = 'n'; % special, tells the graphics to show that cursor is
                % translated currectly but not yet rotated correctly;
            end
            
            if cursorOnTarget && auxInCenter
                state = uint16(CursorStates.STATE_HOVER);
                if holdTimer >= 0
                    holdTimer = int16(0); % reset hold timer -- it could have been nonzero from either previous
                    % target hold or time spent in any tile in Gridlike mode.
                else
                    holdTimer = holdTimer; % allows negative to carry over for selectionRefractoryMS
                end
                
                if lockedParameters.soundOnOverTarget
                    % if we're on autoplay, make a tapping noise
                    lastSoundTime = clock;
                    lastSoundState = uint8(CursorStates.SOUND_STATE_OVER_TARGET);
                end

            elseif stateTimer >= lockedParameters.trialTimeout
                stateTimer = uint16(0);
                state = uint16(CursorStates.STATE_FAIL);
                
            elseif clickTimer >= clickParameters.clickHoldTime && lockedParameters.taskType ~= uint32(cursorConstants.TASK_GRIDLIKE)
       % long enough click to make a selection, and we aren't over the target. Depending on task options, this could cause a failure.
             %  Note that clickTimer has refractory properties                 
                if lockedParameters.falseClickFails
                    % Clicked outside target. FAIL!
                    stateTimer = uint16(0);
                    state = uint16( CursorStates.STATE_FAIL );
                end                
                if lockedParameters.stopOnClick
                    % First undo this time step's velocity->position update,
                    % otherwise the cursor can still move a bit during stop on click.
                    xkRaw(effectorPosInds) = xkRaw(effectorPosInds) - xkMod(effectorVelInds); % seems weird but recall we update raw position using xkMod velocity in updateXk
                    xkMod(effectorPosInds) = xkMod(effectorPosInds) - xkMod(effectorVelInds);
                    % zero velocity due to click.
                    xkMod(effectorVelInds,1) = 0;
                    xkRaw(effectorVelInds,1) = 0;                    
                end
            elseif lockedParameters.taskType ==  uint32(cursorConstants.TASK_GRIDLIKE)
                % GRIDLIKE TASK COUNTING OF TIME SPENT IN WRONG TILE
                % SDS Jan 2016
                if any( currentOccupiedTile )  % to rule out being in no tile
                    if any( currentOccupiedTile ~= previousOccupiedTile )
                        % Entered a new tile - reset timer
                        if holdTimer >= 0
                            holdTimer = int16(0);
                        else
                            holdTimer = holdTimer;
                            % allows negative holdTimer to carry over for selectionRefractoryMS
                        end
                    else % still in same tile as during last tick
                        holdTimer = holdTimer + 1;
                        % still in the same tile as before, so count count up hold timer
                        % note that holdTimer  may never be used for a
                        % time out, but it's doing double duty as a timer
                        % of the when click is allowable again (refractory
                        % period).
                        % taskParams.holdTime should be Inf if
                        % select-via-hold ought to be impossible.
                        if holdTimer > lockedParameters.holdTime
                            % dwelled too long in wrong tile; FAIL!
                            stateTimer = uint16(0);
                            state = uint16(CursorStates.STATE_FAIL);
                        end                      
                    end
                    % We're not on the right tile, and we're on a tile, so
                    % a click at this point ought to incur failure.
                    if clickState == uint16(DiscreteStates.CLICK_MAIN)
                        clickTimer = clickTimer + 1; 
                        if clickTimer >= clickParameters.clickHoldTime
%                             if holdTimer >= 0   % This is what creates the refractory period.
                              % SDS May 2 2017: now that clickTimer is its
                              % own refactory period, above seems unnecessary 
                              state = uint16(CursorStates.STATE_FAIL);
                              stateTimer = uint16(0);
                              if lockedParameters.stopOnClick
                                  % First undo this time step's velocity->position update,
                                  % otherwise the cursor can still move a bit during stop on click.
                                  xkRaw(effectorPosInds) = xkRaw(effectorPosInds) - xkMod(effectorVelInds); % seems weird but recall we update raw position using xkMod velocity in updateXk
                                  xkMod(effectorPosInds) = xkMod(effectorPosInds) - xkMod(effectorVelInds);
                                  % zero velocity
                                  xkMod(effectorVelInds,1) = 0;
                                  xkRaw(effectorVelInds,1) = 0;                                  
                              end
                        end
                    end
                else
                    if holdTimer < 0 % can count up from negative to 0 (being outside of bounday still counts towards grace period.
                        holdTimer = holdTimer + 1;
                    end
                end
            end
            previousOccupiedTile = currentOccupiedTile; % previous tile is set to current tile.      
%% STATE_HOVER
        case {CursorStates.STATE_HOVER}
            % Hover is being over a target when click enabled - Sergey
            stateTimer = stateTimer + 1;
            % SDS Jan 26 2017. I'm making hold to select possible in cursor
            % task, even when click is also an option. Hence, now holdTimer
            % counts up here too.
            % SNF: this doesn't discriminate between dwell and click
            % targets and should be a special case, not the default. In
            % multiclick, the center target is type "dwell" so this doens't
            % muck with the center target's ability to dwell-select. 
           % if ~(lockedParameters.taskType ==  uint32(cursorConstants.TASK_MULTICLICK))
                holdTimer = holdTimer + 1; 
           % end
            % if "stopOffTarget" is false, then we must manually
            %   flag times when cursor is over target to allow click to stop
            allowStop = true;
           
            networkOutput.discrete.send = false;
            % Check whether cursor is in target differs for Gridlike and other keyboard-esque tasks.
            targetColor = 'o'; %could be updated but default = orange
            switch lockedParameters.taskType
                case  uint32(cursorConstants.TASK_GRIDLIKE)
                    myTile = whichGridlikeTile( effectorPos, lockedParameters.gridEdges, lockedParameters.gridTilesEachDim );
                    cursorOnTarget = ~any( myTile ~= currentTargetTile ); % SDS Dec 2016
                case uint32( cursorConstants.TASK_FCC )
                     % closestTargetInd not yet used but could be for selecting specific letters.
                   [cursorOnTarget, closestTargetInd] = FCCisCursorOntarget(effectorPos, cycleIndex, ...
                                                        lockedParameters.targetInds, lockedParameters.numTargets, TASK_DIMS );
               case uint32(cursorConstants.TASK_MULTICLICK) %SNF SEPT
                    %make the cursor color match the instructed click
                    cursorOnTarget = isCursorOnTarget(effectorPos, double(lockedParameters.cursorDiameter)/2, currentTarget, targetRadiusTrans, targetRadiusRot, TASK_DIMS);
                    if (uint16(inputType) == uint16(cursorConstants.INPUT_TYPE_AUTO_ACQUIRE_HS)) || ...
                            (uint16(inputType) == uint16(cursorConstants.INPUT_TYPE_AUTO_ACQUIRE))
                        cursorColors(1:end, 1) = multiClickColors(uint16(currentClickTarg), 1:end); 
                    end
                otherwise
                    cursorOnTarget = isCursorOnTarget(effectorPos, double(lockedParameters.cursorDiameter)/2, currentTarget, targetRadiusTrans, targetRadiusRot, TASK_DIMS);
            end           
            
           % if clickState == uint16(DiscreteStates.CLICK_MAIN)
            if clickState >= uint16(DiscreteStates.CLICK_MAIN) %SNF for multiclick
                clickTimer = clickTimer + 1; 
                if clickTimer >= clickParameters.clickHoldTime % we've clicked for long enough 
                    if holdTimer > 0 % if not in the refractory period.
                        stateTimer = uint16(0); %a different state will be entered no matter what
                        if cursorOnTarget %we clicked while on the target
                            %SNF multiclick: we performed the *correct* click
                            if lockedParameters.taskType == uint32( cursorConstants.TASK_MULTICLICK)
                                if uint16(clickState - 1) == currentClickTarg % this could probably go in the if clickState >= CLICK_MAIN part but let's not rock the boat too hard... yet -SNF
                                    state = uint16(CursorStates.STATE_SUCCESS); %yay
                                else
                                    state = uint16(CursorStates.STATE_FAIL); %boo
                                end
                            else %normal operation: 
                                state = uint16(CursorStates.STATE_SUCCESS); %yay
                            end
                        %   stateTimer = uint16(0);
                        else
                         %   stateTimer = uint16(0);
                            if lockedParameters.falseClickFails %if false clicks are failure, fail. 
                                state = uint16( CursorStates.STATE_FAIL ); %womp womp
                            else                                % otherwise, keep moving and try again
                                state = uint16( CursorStates.STATE_MOVE_CLICK ); % kicked out to move
                            end
                        end
                        
                        if lockedParameters.stopOnClick
                            % First undo this time step's velocity->position update,
                            % otherwise the cursor can still move a bit during stop on click.
                            xkRaw(effectorPosInds) = xkRaw(effectorPosInds) - xkMod(effectorVelInds); % seems weird but recall we update raw position using xkMod velocity in updateXk
                            xkMod(effectorPosInds) = xkMod(effectorPosInds) - xkMod(effectorVelInds);
                            % zero velocity due to click.
                            xkMod(effectorVelInds,1) = 0;
                            xkRaw(effectorVelInds,1) = 0;
                         end
                    end
                end
                
            elseif ~cursorOnTarget || ~auxInCenter
                % the elseif means that if mid-click and drifting off a
                % target, that's not yet a fail. But if NOT still clicking,
                % and drift off a target, then it goes to STATE_MOVE_CLICK.
                % Note that due to logic above in the click check, gridlike
                % task is less forgiving.
                state = uint16(CursorStates.STATE_MOVE_CLICK);%SNF bug-check: shouldn't the state get reset to 0 here? Jan 30 2019
                % we were over the target, but now we're not, so either
                % left target or the tile (gridlike). Either way, hold timer becomes zero if nonnegative/
                if holdTimer > 0 % rapidly fluttering over target in gridlike task doesn't nullify refractory period.
                    holdTimer = int16(0);
                end
            % the following condition should probably not be the default, or should have a flag like "holdBackstop"    
          %  elseif ~(lockedParameters.taskType ==  uint32(cursorConstants.TASK_MULTICLICK))...
          %              && holdTimer >= lockedParameters.holdTime
            elseif  holdTimer >= lockedParameters.holdTime
                % held over the target long enough to acquire it
                % we do not want this to happen if it's closed loop multiclick
                if ~((lockedParameters.taskType ==  uint32(cursorConstants.TASK_MULTICLICK)) &&...
                        ((uint16(inputType) == uint16(cursorConstants.INPUT_TYPE_CURSOR_HEADSTILL)) ||...
                         (uint16(inputType) == uint16(cursorConstants.INPUT_TYPE_DECODE_V))))
                    acquireTime = stateTimer;
                    stateTimer = uint16(0);
                    state = uint16(CursorStates.STATE_SUCCESS);
                    holdTimer = int16(0);
                end
            end 
            %separating this out because it's always going to overrule the
            %rest of the cases: 
            if stateTimer >= lockedParameters.trialTimeout
                stateTimer = uint16(0);
                state = uint16(CursorStates.STATE_FAIL);
                holdTimer = int16(0);  % should be clickTimer
            %else
%                 clickTimer = int16(0);              
                % likely redundant to check at top of the function, but
                % can't hurt here.
            end
%% STATE_ACQUIRE
        case {CursorStates.STATE_ACQUIRE} % This means cursor is over the target when dwell (not click) is the selection mode.
            stateTimer = stateTimer + 1;
            holdTimer = holdTimer + 1;
            % if "stopOffTarget" is false, then we must manually
            %   flag times when cursor is over target to allow click to stop
            % Check whether cursor is in target differs for Gridlike task.
            switch lockedParameters.taskType
                case  uint32(cursorConstants.TASK_GRIDLIKE)
                    myTile = whichGridlikeTile( effectorPos, lockedParameters.gridEdges, lockedParameters.gridTilesEachDim );
                    cursorOnTarget = ~any( myTile ~= currentTargetTile ); % SDS Dec 2016
                    targetColor = 'o'; % in Gridlike task, it's orange during hold
                otherwise
                    cursorOnTarget = isCursorOnTarget(effectorPos, double(lockedParameters.cursorDiameter)/2, currentTarget, targetRadiusTrans, targetRadiusRot, TASK_DIMS);
                    targetColor = 'o'; % in other task variants, target also organe during hold
            end
            
            allowStop = true;
            
            if ~cursorOnTarget || ~auxInCenter
                state = uint16(CursorStates.STATE_MOVE);
                if holdTimer > 0
                    % check for > 0 so briefly entering and exiting a
                    % target doesn't void negative holdTime that is used as
                    % a refractory period.
                    holdTimer = int16(0);
                end
            elseif holdTimer >= lockedParameters.holdTime
                acquireTime = stateTimer;
                stateTimer = uint16(0);
                state = uint16(CursorStates.STATE_SUCCESS);
            end
%% STATE_SUCCESS
        case {CursorStates.STATE_SUCCESS}
            stateTimer = stateTimer + 1;
            inputType = lockedParameters.inputType;
            trialNum = trialNum+1;
            
            % how do we score this trial?
            localTotal = localTotal+1;
            localAcquired = localAcquired + 1;
            localTotalTime = localTotalTime + acquireTime;
            
            localAcqTime = uint16(single(localTotalTime) / single(localTotal));
            lastAcquireSuccess = true;
            
            if lockedParameters.soundOnSuccess && stateTimer <= 1
                lastSoundTime = clock;               
                lastSoundState = uint8(CursorStates.SOUND_STATE_SUCCESS);
            end

            if lockedParameters.showScores && localTotal == lockedParameters.trialsPerScore
                stateTimer = uint16(0);
                state = uint16(CursorStates.STATE_SCORE_PAUSE);
                totalScore = totalScore + localScore;
            else
                stateTimer = uint16(0);
                state = uint16(CursorStates.STATE_PRE_TRIAL);
            end
            % if we've finished a cycle, start a new cycle ("chain" in rigC parlance). 
            % SDS Dec 2016, trying to make sense of this.
            % cycleIndex tracks where in the cycle we are. So e.g. if there's an
            % 8 target cycle, we might do ~5 cycles in a block (40 trials).
            % cycleIndex will range from 1 to 8.
            % targetInds has the coordiantes of targets, it is set in the
            % parameter scripts. numTargets is e.g. 8 (for 8 Target Task),
            % and is also set in the parameter script.
            switch lockedParameters.taskType
                case {uint32(cursorConstants.TASK_PINBALL)}
                    if ~mod(trialNum-1, lockedParameters.numTargets)
                        cycleNum = cycleNum+1;
                        % randomize the order of targets for the next cycle.
                        targetOrder(1:lockedParameters.numTargets) = randperm(lockedParameters.numTargets);
                    end
                    cycleIndex = mod(trialNum-1, lockedParameters.numTargets)+1;
                case {uint32(cursorConstants.TASK_GRIDLIKE), uint32(cursorConstants.TASK_RANDOM) }
                    % Gridlike-task and Random task have no cycles, since each next target
                    % is always random after fail or success (there aren't
                    % a set of targets to get through).
                case uint32(cursorConstants.TASK_CENTER_OUT_NO_BACK)
                    if lockedParameters.discreteOLMode
                        if ~mod(trialNum-1, lockedParameters.numTargets-1)
                            cycleNum = cycleNum+1;
                            % randomize the order of targets for the next cycle.
                            targetOrder(1) = targetOrder(lockedParameters.numTargets);
                            targetOrder(2:lockedParameters.numTargets) = randi(lockedParameters.numTargets,lockedParameters.numTargets-1,1);
                        end
                        cycleIndex = mod(trialNum-1, lockedParameters.numTargets-1)+1;
                    else
                        if ~mod(trialNum-1, lockedParameters.numTargets)
                            cycleNum = cycleNum+1;
                            % randomize the order of targets for the next
                            % cycle.
                            targetOrder(1:lockedParameters.numTargets) = randperm(lockedParameters.numTargets);
                        end
                        cycleIndex = mod(trialNum-1, lockedParameters.numTargets)+1;
                    end   
                case {uint32(cursorConstants.TASK_CENTER_OUT), uint32(cursorConstants.TASK_MULTICLICK)}
                    if ~mod(trialNum-1, lockedParameters.numTargets*2)
                        cycleNum = cycleNum+1;
                        % Randomize the order of targets for the next cycle.
                        targetOrder(1:lockedParameters.numTargets) = randperm(lockedParameters.numTargets);
                    end
                    cycleIndex = uint16(floor(mod(double((trialNum-1)/2), lockedParameters.numTargets)))+1;
            end           
%% STATE_FAIL
        case {CursorStates.STATE_FAIL}
            stateTimer = stateTimer+1;
            lastAcquireSuccess = false;
            % Check whether cursor is in target differs for Gridlike task.
            switch lockedParameters.taskType
                case  uint32( cursorConstants.TASK_GRIDLIKE )
                    myTile = whichGridlikeTile( effectorPos, lockedParameters.gridEdges, lockedParameters.gridTilesEachDim );
                    cursorOnTarget = ~any( myTile ~= currentTargetTile ); % SDS Dec 2016
                case uint32( cursorConstants.TASK_RAYS )
                    targetColor = 'r'; % makes it so target is flashed red to indicate what selection was made.
                otherwise %why are we even checking this? -SF Jan 2019
                    cursorOnTarget = isCursorOnTarget(effectorPos, double(lockedParameters.cursorDiameter)/2, currentTarget, targetRadiusTrans, targetRadiusRot, TASK_DIMS);
            end
            
            if stateTimer >=  lockedParameters.failurePenalty
                trialNum = trialNum + 1;
                stateTimer = uint16(0);
                % how do we score this trial?
                localTotal = localTotal+1;
                localAcqTime = uint16(single(localTotalTime) / single(localTotal));
                if lockedParameters.showScores && localTotal == lockedParameters.trialsPerScore
                    state = uint16(CursorStates.STATE_SCORE_PAUSE);
                    totalScore = totalScore + localScore;
                else
                    state = uint16(CursorStates.STATE_PRE_TRIAL);
                end                
                %% if doing center out no back, cycle to next target instead
                %of repeating the failed one (FRW)
                switch lockedParameters.taskType
                    case uint32(cursorConstants.TASK_CENTER_OUT_NO_BACK)
                        if ~mod(trialNum-1, lockedParameters.numTargets)
                            cycleNum = cycleNum+1;
                            targetOrder(1:lockedParameters.numTargets) = randperm(lockedParameters.numTargets);
                        end
                        cycleIndex = mod(trialNum-1, lockedParameters.numTargets)+1;
                end
            end
            if lockedParameters.soundOnFail && stateTimer <= 0 % second condition is so failure sound played just once
                lastSoundTime = clock;
                lastSoundState = uint8(CursorStates.SOUND_STATE_FAIL);
            end      
%% STATE_END
        case {CursorStates.STATE_END}            
            stateTimer = stateTimer + 1;
            % Hide the target so it's clear to participant that the task is
            % complete.
            % Added SDS Jan 2017
            currentTarget(1:end) = 9999; 
            % If this is gridlike task, also update the
            % currentTargetTile
            if lockedParameters.taskType == uint32(cursorConstants.TASK_GRIDLIKE)
                currentTargetTile = uint16(zeros([double(xkConstants.NUM_TARGET_DIMENSIONS) 1])); % all zeros means not active
            end            
%% STATE_SCORE_PAUSE % Not used now  - SDS Dec 2016 %SF sees it being called if we score tasks Jan 2019
        case {CursorStates.STATE_SCORE_PAUSE}
            stateTimer = stateTimer + 1;
            if stateTimer >= SCORE_LENGTH
                state = uint16(CursorStates.STATE_SCORE_TARGET);
                stateTimer = uint16(0);
                currentTarget = single(zeros( double(xkConstants.NUM_TARGET_DIMENSIONS),1)); 
            end
%% These states are all unused:             
% %% STATE_SCORE_TARGET       
%         % Not used now  - SDS Dec 2016
%         case {CursorStates.STATE_SCORE_TARGET}
%             stateTimer = stateTimer + 1;
%             if isCursorOnTarget(effectorPos, double(lockedParameters.cursorDiameter)/2, currentTarget, targetRadiusTrans, targetRadiusRot, TASK_DIMS);
%                 state = uint16(CursorStates.STATE_PRE_TRIAL);
%                 stateTimer = uint16(0);
%                 localTotal = uint16(0);
%                 localAcquired = uint16(0);
%                 localTotalTime = uint16(0);
%             end
% %% STATE_CENTER_TARGET
%         case {CursorStates.STATE_CENTER_TARGET}
%             stateTimer = stateTimer + 1;
%             initialFingerPosition=mouse(1:2);
%             initialCursorPosition = single( effectorPos ); % the (1:NUM_DIMS) is to handhold compilter about the dimensionality
%            
%             %gridlike, FCC, RAYS, variants never enters this state
%             
%             if isCursorOnTarget(effectorPos, double(lockedParameters.cursorDiameter)/2, currentTarget, targetRadiusTrans, targetRadiusRot, TASK_DIMS)
%                 state = uint16(CursorStates.STATE_SUCCESS);
%                 stateTimer = uint16(0);
%             end      
% %% STATE_FINGER_MOVED
%         % Not currently used. -SDS Dec 2016
%         case {CursorStates.STATE_FINGER_MOVED}
%             if ~fingerOffTarget
%                 stateTimer = uint16(0);
%                 state = uint16(CursorStates.STATE_FAIL);
%                 inputType = previousInput;
%             end           
%% %%%%%%%%%%%%%%%% END STATE MACHINE %%%%%%%%%%%%%%%%%%%%%%%%%%%%%%%%%%%%%     
    end 
%% %%%%%%%%%%%%%%%%%%%%%%%%%%%%%%%%%%%%%%%%%%%%%%%%%%%%%%%%%%%%%%%%%%%%%%%%
end

if lockedParameters.maxTaskTime && totalTaskTime > lockedParameters.maxTaskTime
    state = uint16(CursorStates.STATE_END);
end

taskOutput.xk = xkRaw; % feed *raw* xk back out, which goes to decoder and file logger
taskOutput.currentTarget = single(currentTarget(:,1));
taskOutput.state = state;
taskOutput.clickTarget = uint16(currentClickTarg); %SF: sure hope this doesn't destroy anything
taskOutput.taskType = uint16(lockedParameters.taskType); %SNF added for multiclick checking 
% make sure we send the compiled dimension size, but only fill the used task ones.
cursorPosition = single(effectorPos');
cursorVelocity = single(effectorVel');
taskAgnosticVel = single(taskAgnosticXk(effectorVelInds)');
prevClickState = clickState; %update for the next loop -SNF
%% PACK DATA FOR UDP OUTPUT (filelogger continuous)
taskOutput.continuous = packFileLoggerFormatAndData('continuous', ...
    TASK_NAME, VERSION_ID, ...
    'clock', clock, ...
    'pause', pauseTriggered, ...
    'xpcRequestClock', behaviorRequestClock, ...
    'peripheralTimestamp', peripheralTimestamp, ...
    'state', state, ...
    'inputType', inputType, ...
    'windowsPacketSize', behaviorPacket.windowsPacketSize, ...
    'windowsMousePosition', behaviorPacket.windowsMousePosition, ...
    'windowsTimestamp', behaviorPacket.windowsTimestamp, ...
    'windowsPC1GazePoint', behaviorPacket.windowsPC1GazePoint, ...
    'windowsPC1GazePointValid', behaviorPacket.windowsPC1GazeValid, ...
    'rigidBodyPosXYZ', behaviorPacket.rigidBodyPosXYZ, ...
    'rigidBodyRotXYZ', behaviorPacket.rigidBodyRotXYZ, ...
    'windowsPC1Timestamp', behaviorPacket.windowsPC1Timestamp, ...
    'xpcScreenUpdateClock',vizPacket.xpcScreenUpdateClock,...
    'cursorPosition', cursorPosition(1:NUM_DIMS), ...
    'currentTarget', single(currentTarget(:,1)), ...
    'currentTargetType', uint16(currentTargetType),...
    'clickTarget', uint16(currentClickTarg),... %SNF multiclick, added March 2019
    'clickState', uint16(clickState),...
    'xk', single(taskOutput.xk),...
    'stateTimer', stateTimer, ...
    'holdTimer', holdTimer, ...   
    'fingerLifted',uint8(fingerLifted),...
    'behaviorPacketSize', behaviorPacket.packetSize, ...
    'xpcTET', single(xpcTET), ...
    'robotTimestamp', behaviorPacket.robotTimestamp, ...
    'robotPosition', robotPosition, ...
    'clickTimer', clickTimer, ... % DEV, keep around for now while there's space as it could be helpful
    ...'currentOccupiedTile', currentOccupiedTile, ... % For Gridlike task Added 15 Dec 2016 SDS %SNF commented out March 2019
    'gain', cursorParameters.gain, ...  % not locked  
    'powerGain', cursorParameters.powerGain, ...
    'powerGainUnityCrossing', cursorParameters.powerGain, ...
    'cursorPosition2', cursorPosition2(1:NUM_DIMS), ... % For RAYS only, not essential since can eb reconstructed from cursorPosition SDS May 2017
    'xkModBiasEst', single(xkModBiasEst) ... %the bias estimate coming from the bias killer that acts on xkMod (after nonlinear gain)
    );
    %'windowsPC1HeadRot', behaviorPacket.windowsPC1HeadRot, ...
    %'windowsPC1HeadRotValid', behaviorPacket.windowsPC1HeadRotValid, ...
% 'windowsPC1TobiiTimestamp', behaviorPacket.windowsPC1TobiiTimestamp, ...
%'taskAgnosticVel', taskAgnosticVel(1:NUM_DIMS), ...
% prepare some additional info for gridlike task.
gridExtrema = max( lockedParameters.gridEdges );  % assume symmetry, record just max edge to save space
% Send these all together to conserve bytes, because the names are all encoded too.
% DIMENSION-DEPENDENT [flag for me, search for it when increasing dimensionality]
workspaceAll = [lockedParameters.workspaceX; 
    lockedParameters.workspaceY;
    lockedParameters.workspaceZ;
    lockedParameters.workspaceR;
    lockedParameters.workspaceR2];
% added SDS Jan 2016
%% SEND DISCRETE DATA TO FILELOGGER
taskOutput.discrete = packFileLoggerFormatAndData('discrete', ...
    TASK_NAME, VERSION_ID, ...
    'clock', clock,...
    'blockNumber', stateParameters.blockNumber,...
    'taskType', lockedParameters.taskType, ...
    'targetDiameter', single( targetRadiusTrans*2 ), ...
    'trialDelayLength', trialDelayLength, ...
    'currentTarget', currentTarget,...
    'speedCode', speedCode,... %for instructed speed experiments
    'wiaCode', wiaCode,... %for WIA-type experiments
    ...'cycleIndex', cycleIndex,... % Not strictly necessary but maybe useful. Remove if space is needed %removed SNF March 2019
    'currentTargetType', uint16(currentTargetType),...
    'nextTargetType', uint16(nextTargetType),... %SNF multiclick
    'holdTime', lockedParameters.holdTime, ...
    'clickPercentage', single(lockedParameters.clickPercentage), ...
    'hmmClickLikelihoodThreshold',clickParameters.hmmClickLikelihoodThreshold,...
    'clickHoldTime', clickParameters.clickHoldTime, ...
    'clickSource', clickParameters.clickSource, ...% used for training click so we always need this 
    'trialNum', trialNum, ...
    'inputType', inputType, ...
    'workspace', workspaceAll, ...    
    'recenterOnSuccess', lockedParameters.recenterOnSuccess,...
    'recenterOnFail', lockedParameters.recenterOnFail,...
    'recenterDelay', lockedParameters.recenterDelay,...
    'errorAssistR',single(lockedParameters.errorAssistR),...    
    'errorAssistTheta',single(lockedParameters.errorAssistTheta),...
    'errorAssistAxis',single(lockedParameters.errorAssistAxis),... % added Oct 27 2016 SDS
    'hmmClickSpeedMax',single(clickParameters.hmmClickSpeedMax),...
    'outputType', outputType, ...
    'xk2EffectorPosInds', uint8(effectorPosInds(1:NUM_DIMS)), ...  % want to know hor state is being mapped to game horizontal, veritacl, depth, rotate, ...
    ... %'xk2EffectorVelInds', uint8(effectorVelInds(1:NUM_DIMS)), ... %removed by SF Feb 2019
    ...'currentTargetTile', uint8(currentTargetTile), ... % for Gridlike task Added Dec 15 2016 SDS %commented out SNF March 2019
    'selectionRefractoryMS', uint16( lockedParameters.selectionRefractoryMS ), ... % for Gridlike task Added Dec 15 2016 SDS
    ...'gridExtrema', single( gridExtrema ), ... %commented out SNF March 2019
    ...'gridTilesEachDim', uint8( lockedParameters.gridTilesEachDim ), ...%commented out SNF March 2019
    'numTargets',  uint16( lockedParameters.numTargets ), ...  % used for RAYS bitrate compute   
    'targetRotDiameter', single( targetRadiusRot*2 ), ...'
    'nextClickTarg', uint16( nextClickTarg)... %SNF multiclick - use the upcoming one that gets set at the beginning of each trial 
);
% SDS Removed Dec 2016 because we're up against the packet size and they're
% not currently used:
%     'state', state, ...   %this is saved in continuous so why was it here?
%     'gloveBias', lockedParameters.gloveBias, ...
%     'mouseOffset', lockedParameters.mouseOffset, ...
%    'nextTarget', currentTarget,...
%    'useRandomDelay', lockedParameters.useRandomDelay, ...
% xk2HorizontalPos = uint8( lockedParameters.xk2HorizontalPos );
% xk2VerticalPos = uint8( lockedParameters.xk2VerticalPos );
% xk2HorizontalVel = uint8( lockedParameters.xk2HorizontalVel );
% xk2VerticalVel = uint8( lockedParameters.xk2VerticalVel );
% xk2DepthPos = uint8( lockedParameters.xk2DepthPos );
% xk2DepthVel = uint8( lockedParameters.xk2DepthVel );
% xk2RotatePos = uint8( lockedParameters.xk2RotatePos );
% xk2RotateVel = uint8( lockedParameters.xk2RotateVel );
% removed to save space , currently unused
%    'useGloveLPF', uint8(lockedParameters.useGloveLPF),...
%    'useMouseLPF', uint8(lockedParameters.useMouseLPF),...
%    'gloveThreshold', clickParameters.gloveThreshold, ...
%    'gloveIndices', clickParameters.gloveIndices, ...
%    'gloveYCorrection', single(lockedParameters.gloveYCorrection), ...
%    'gloveXCorrection', single(lockedParameters.gloveXCorrection), ...
%    'initialFingerPositon',initialFingerPosition,...
%    'fingerPositionTolerance',single(cursorParameters.fingerPositionTolerance),...
%% SEND DATA OUT TO VIZ
upcomingTarget = single(zeros(2,1));
if lockedParameters.discreteOLMode
    upcomingTarget = lockedParameters.targetInds(1:2,targetOrder(cycleIndex+1));
else
    upcomingTarget(:) = single(-1);
end
taskOutput.screen = packFileLoggerFormatAndData('screen', ...
    TASK_NAME, VERSION_ID, ...
    'clock', clock,...
    'totalTaskTime',totalTaskTime,...
    'blockNumber', stateParameters.blockNumber,...
    'state',state,...
    'cursorPosition',  horzcat(cursorPosition(1:NUM_DIMS)', cursorPosition2(1:NUM_DIMS)', cursorPosition3(1:NUM_DIMS)),... % handhold the compiler with dims here
    'cursorColors', cursorColors,...
    'currentTarget', currentTarget,...
    'upcomingTarget', upcomingTarget,...
    'cursorDiameter', lockedParameters.cursorDiameter,...
    'targetDiameter', single( targetRadiusTrans*2 ),...
    'targetRotDiameter', single( targetRadiusRot*2) ,...
    'targetColor', targetColor, ...
    'localAcquired', localAcquired,...
    'localTotal', localTotal,...
    'localAcqTime', localAcqTime,...
    'inputType', inputType,...
    'speedCode', speedCode,...
    'wiaCode', wiaCode,...
    'drawNumbersOnTargets',lockedParameters.drawNumbersOnTargets,...
    'showWiaText',lockedParameters.showWiaText,...
    'nextClickTarg',  nextClickTarg,... %SNF multiclick - use the upcoming one that gets set at the beginning of each trial
    'taskType', lockedParameters.taskType,...
    'recenterDelay', lockedParameters.recenterDelay,...
    'cursorVelocity', cursorVelocity(1:NUM_DIMS), ...
    'outputType', outputType, ...
    'numDisplayDims', lockedParameters.numDisplayDims, ...
    'showXYZaura', lockedParameters.showXYZaura, ... % not logged.
    'displayObject', lockedParameters.displayObject, ... % not logged
    'numTargets',uint8(lockedParameters.numTargets), ... % used only by PTB
    'nextTarget', nextTarget(1:2),...
    'targetInds', int16(lockedParameters.targetInds(1:2,1:32)), ... % only twoD, 8 targets, to support doing monthly R8/Fitts in PTB from same compiled code.
    'cursorAlpha2', cursorAlpha2, ... % only used for RAYS to shade cursor2.
    'splitDimensions', lockedParameters.splitDimensions, ... % instructs whether to render graphics as two cursors with half as many DOF
    'gain', cursorParameters.gain ... % SDS April 24 2018 added so Darrel can read this.
);
% removed because I don't think it makes sense to send these to screen in >
% 2D. 
% targetInds is HUGE, we'd only want to send it for the 2D, PTB engine
% where we actualy drew all the possible targets on the screen.
% care, I think. nextTarget isn't used by screen either.
%     'targetInds',int16(lockedParameters.targetInds(1:int8(xkConstants.NUM_TARGET_DIMENSIONS),1:uint8(cursorConstants.MAX_TARGETS))), ...  % SDS Aug 2016: uses a fair number of bytes, lower if running out
%% SEND DATA OUT TO SOUND
taskOutput.sound = packFileLoggerFormatAndData('screen', ...
    TASK_NAME, VERSION_ID, ...
    'clock', clock,...
    'vizState',state,...
    'lastSoundTime',lastSoundTime,...
    'lastSoundState',lastSoundState,...
    'wiaCode',wiaCode...
    );
%% SET SEND FLAGS FOR NETWORK OUTPUTS
if(clock < INIT_TIME)
    taskOutput.discrete.data.send = false;
    taskOutput.continuous.data.send = false;
    taskOutput.screen.data.send = false;
    taskOutput.sound.data.send = false;
    
    if(mod(clock, 10)==0)
        taskOutput.sendFormat = true;
    else
        taskOutput.sendFormat = false;
    end
    stateTimer = uint16(0);
else
    taskOutput.discrete.data.send = writeDiscreteData;
    taskOutput.continuous.data.send = writeContinuousData;
    taskOutput.screen.data.send = true;
    taskOutput.sound.data.send = true;
    taskOutput.sendFormat = false;
    taskOutput.inputType = inputType;
end
taskOutput.wiaCode = wiaCode;
taskOutput.speedCode = speedCode;
taskOutput.paused = pauseTriggered;
taskOutput.allowStop = allowStop;
lastState = state;

end

function vizPacket = parseVizPacket(packetData)

    vizPacket.xpcScreenUpdateClock = typecast(packetData(28+[1:4]), 'uint32');

end

function vizPacket = initVizPacket()

    vizPacket.xpcScreenUpdateClock = uint32(0);

end

function [icot, translateOnTarget] = isCursorOnTarget(effectorPos, cursorRadius, targetPosition, targetRadius, targetRotRadius, TASK_DIMS)
    % Effective April 4 2017, dims 1:4 (so including rotation) are treated
    % the same, meaning that cursor needs to be within hyperradius. It is
    % highly advised to NOT use XYZ aura in the mode, as it is misleading.
    %
    % Effective Feb 28 2017, the cursor radius no longer "matters", i.e.
    % it's not used for isCursorOnTarget calculation. Only the target
    % radius matters. This makes tasks effectively harder, but also removes
    % a potential confusion point. Now that the target isn't a sphere
    % anyway, the boundary isn't visually marked anyway so this seems more
    % principled.
    % boundary checking for dims 4+ will be handled separately for the 3d
    % translational dimensions
    %
    % translateOnTarget returns true if at least the translation (dims 1:3)
    % are over the target. This can be used to visually depict that
    % translation, but not rotation, is correct. - SDS March 2017
%     if TASK_DIMS > 4
%         useDims = uint8(3); 
%     else
        useDims = TASK_DIMS;
%     end

    if sqrt( sum( ((double( effectorPos(1:useDims) ) - double( targetPosition(1:useDims) )).^2 ) ) ) < ...
            double(targetRadius)
        translateOnTarget = true;
        % Translation check passed
%         if TASK_DIMS >= 5
%             % Are we within the rotational radius hypersphere?
% %             if sqrt( sum((double( effectorPos(5:TASK_DIMS) ) - double( targetPosition(5:TASK_DIMS) )).^2 ) ) < ...
%             if sqrt( sum((double( effectorPos(4:TASK_DIMS) ) - double( targetPosition(4:TASK_DIMS) )).^2 ) ) < ...
%                     double( targetRotRadius ) 
%                 icot = true;
%             else
%                 icot = false;
%             end       
%         else
            icot = true;
%         end
    else
        icot = false;
        translateOnTarget = false;
    end
end

function [selectionHappens, cursorOnCorrectTarget, closestTargetInd] = RAYSselection(effectorPos, selectionRadius, currentTargetInd, ...
                        targetInds, numTargets, TASK_DIMS )
    % The key logic for RAYS is implemented here. When cursor is far enough
    % from origin, selection is whichever target its angle closest to.
    % INPUTS:
    %   effectorPos        cursor position Nx1
    %   selectionRadius    how far from origin triggers selection
    %   currentTargetInd   index into <targetInds> for which target is active
    %   targetInds         Nx cursorConstants.MAX_TARGETS of target coordinates
    %   numTargets         How many of targetInds are valid in this task.
    %   TASK_DIMS          How many of the possible target dimensions are in use
    %                    in this task.
    % OUTPUTS:
    %   cursorOnAnyTarget  boolean, true if any targets are selected (i.e.
    %                      cursor is beyond selectionRadius
    %   cursorOnCorrectTarget  whether cursor is currently closest to correct
    %                      target (reproted even if cursorOnAnyTarget is
    %                      false).
    %   closestTargetInd   index into which target cursor is closest to.
    %                      (reproted even if cursorOnAnyTarget is
    %                      false).
    %
    
    
    % Which target ind am I closest to?
    allDiffs = repmat( effectorPos(1:TASK_DIMS), 1, numTargets ) - targetInds((1:TASK_DIMS),1:numTargets);
    allDists = sqrt( sum( allDiffs.^2, 1) );
    [~, closestTargetInd] = min( allDists );
    cursorOnCorrectTarget =  closestTargetInd == currentTargetInd;
    % for iTarg = 1: numTargets
    %
    % end
    
    % Has cursor crossed the selection border?
    selectionHappens = norm( effectorPos(1:TASK_DIMS) ) >= selectionRadius;
end

function [isCursorOnTarget, closestTargetInd] = FCCisCursorOntarget(effectorPos, currentTargetInd, ...
                        targetInds, numTargets, TASK_DIMS )
    % The key logic for FCC keyboard is implemented here. Looks at what
    % target is closest in XYZ, and then, within those, which radial option
    % it is closest to.
    %
    % INPUTS:
    %   effectorPos        cursor position Nx1
    %   currentTargetInd   index into <targetInds> for which target is active
    %   targetInds         Nx cursorConstants.MAX_TARGETS of target coordinates
    %   numTargets         How many of targetInds are valid in this task.
    %   TASK_DIMS          How many of the possible target dimensions are in use
    %                      in this task (not currently used).
    % OUTPUTS:
    %   isCursorOnTarget   boolean, true if correct target is selected.
    %
    %   closestTargetInd   index into which target cursor is closest to.
    %                      (reproted even if cursorOnAnyTarget is
    %                      false).
    if TASK_DIMS >= 3 % makes it a bit more robust to lowD use if for whatever
                      % reason we do that
        spatialDims = uint8(3);
        rotDims = uint8(4);
    else
        spatialDims = TASK_DIMS;
        rotDims = uint8([]); % Shouldn't happen.
    end
    
    % Which SPATIAL target index am I closest to?
    allDiffs = repmat( effectorPos(1:spatialDims), 1, numTargets ) - targetInds((1:spatialDims),1:numTargets);
    allDists = sqrt( sum( allDiffs.^2, 1) );
    closestDistance = min( allDists );
    % No
    EPS = 1e-7;
    % what are the target inds that I'm closest to. I use EPS so that tiny numerical 
    % differences won't cause one to be mised out.
    possibleTargets = find( allDists <= (closestDistance + EPS) );
    % now see which of these spatial closests the cursor is closest to in 
    % the rotational DOF.
    rotDiffs = targetInds(rotDims,possibleTargets) - repmat( effectorPos(rotDims), 1, numel( possibleTargets ) );
    rotDists = sqrt( sum( rotDiffs.^2, 1) );
    [~, closestRotInd] = min( rotDists );
    closestTargetInd = possibleTargets(closestRotInd);
    isCursorOnTarget =  closestTargetInd == currentTargetInd;
end

function eachDimTile = whichGridlikeTile( effectorPos, gridEdges, tilesEachDim )
    % This function is used during the 'gridlike' mode of the cursorTask.
    % It computes, based on the position of the effector, which 'tile' that
    % the high-dimensional 'grid' has been partitioned into the effector is
    % currently in. This is returned as <eachDimTime>, a set of tile coodinates, one for
    % each (active) dimension of the task. Tile coordinates correspond to
    % edges (again in each active dimension) of each tile, which is in
    % <gridEdges>.
    % returning all zeros means effector is not in any of the tiles.
    % Sergey Stavisky Dec 13 2016
    
    % TODO: Adapt for >= 4D
    eachDimTile = uint16( zeros( size( tilesEachDim ) ) );
    for iDim = 1 : numel( effectorPos ) % loop across dimensions. Sizing by effectorPos makes it robust to this dim being smaller than tilesEachDim, gridEdges (which are sized to max allocated)
        if tilesEachDim(iDim) > 0
            
            % Which tile am I in?            
            myTile = find( ( effectorPos(iDim) > gridEdges(1:tilesEachDim(iDim),iDim) ) & ...
                ( effectorPos(iDim) <= gridEdges(2:tilesEachDim(iDim)+1,iDim) ) );
            if isempty( myTile )
                % not in any tile for this dimension, which means not in
                % any tiles
                eachDimTile = uint16( zeros( size( tilesEachDim ) ) );
                break                
            else
                eachDimTile(iDim) = myTile;
            end
        else
            % do nothing, nextTarget(iDim) stays how it
            % was initialized, presumably 0
        end
    end
end
